simulink model "Exercicio_1f_sim"  (R2016a)
settings: Solver=VariableStepAuto  StartTime=0.0  StopTime=t_sim  RelTol=1e-3
values from neighbouring files (symbols this model uses):
  A = [[0,1,0];[0,0,1];[-0.005,-0.11,-0.7]]    [Exercicio_1.m]    (also in matlab.mat = [0  1  0; 0  0  1; -0.005  0.11  -0.7])
  A2 = [[-0.2,-0.2,0.4];[0.5,0,1];[0,-0.4,-0.4]]    [Exercicio_1.m]    (also in matlab.mat = [-0.2  -0.2  0.4; 0.5  0  1; 0  -0.4  -0.4])
  A_AObs = (A_Abb-(A_Ke*A_Aab))    [Exercicio_1.m]    (also in Exercicio_1_teste.m)
  A_BObs = ((A_AObs*A_Ke) + A_Aba - (A_Ke*A_Aaa))    [Exercicio_1.m]    (also in Exercicio_1_teste.m = ((A_AObs*Ke) + A_Aba - (A_Ke*A_Aaa)))
  A_CObs = [[0 0];[eye(2)]]    [Exercicio_1.m]    (also in Exercicio_1_teste.m = (eye(2)))
  A_DObs = [1;A_Ke]    [Exercicio_1.m]    (also in Exercicio_1_teste.m)
  A_FObs = (A_Bb - (A_Ke*A_Ba))    [Exercicio_1.m]    (also in Exercicio_1_teste.m)
  A_K_cntrl = acker(A,B, p_mf)    [Exercicio_1.m]
  B = [[0.1];[-0.2];[-0.1]]    [Exercicio_1.m]    (also in matlab.mat = [0.1 -0.2 -0.1])
  B2 = [[0.01];[0];[0.05]]    [Exercicio_1.m]    (also in matlab.mat = [0.01 0 0.05])
  B_AObs = (B_Abb-(B_Ke*B_Aab))    [Exercicio_1.m]
  B_BObs = ((B_AObs*B_Ke) + B_Aba - (B_Ke*B_Aaa))    [Exercicio_1.m]
  B_CObs = [[0 0];[eye(2)]]    [Exercicio_1.m]
  B_DObs = [1;B_Ke]    [Exercicio_1.m]
  B_FObs = (B_Bb - (B_Ke*B_Ba))    [Exercicio_1.m]
  B_K_cntrl = acker(A2,B2, p_mfB)    [Exercicio_1.m]
  C = [0,0,1]    [Exercicio_1.m]    (also in matlab.mat = [0 0 1])
  C2 = [1,0,0]    [Exercicio_1.m]    (also in matlab.mat = [1 0 0])
  D = [0]    [Exercicio_1.m]    (also in matlab.mat = 0)
  D2 = [0]    [Exercicio_1.m]    (also in matlab.mat = 0)
  N_termo_A1f = rscale(AreordA,AreordB,AreordC,D,A_K_cntrl)    [Exercicio_1.m]
  N_termo_B1f = rscale(Breord,B2,C2,D2,B_K_cntrl)    [Exercicio_1.m]
settings Model: Creator=Usuario  LastModifiedBy=Eletrônica Auto Poli

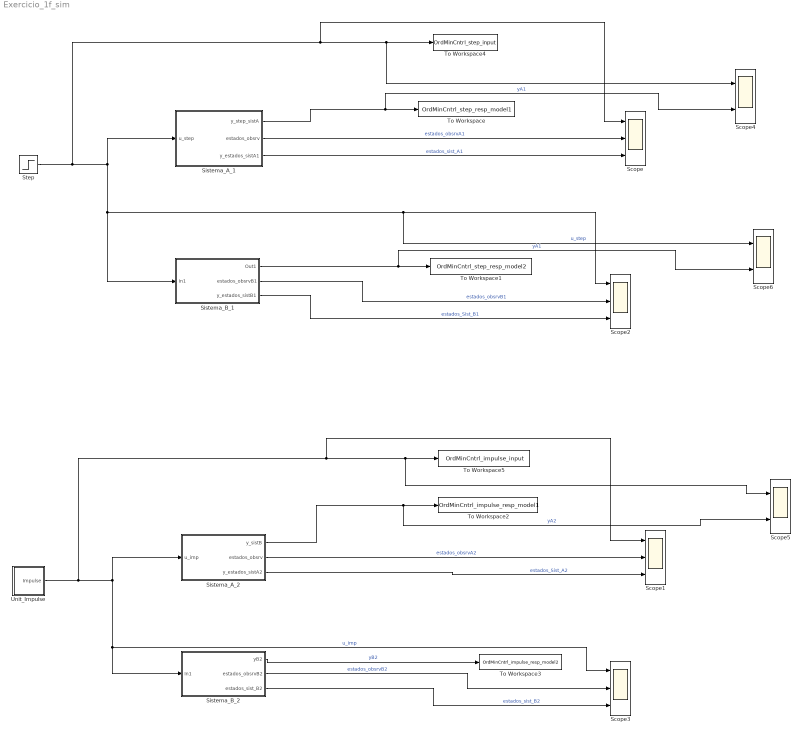
== system Exercicio_1f_sim ==
  Scope{,1..3} (4 alike) : Scope  NumInputPorts=3
  Scope4 : Scope  NumInputPorts=2
  Scope5 : Scope  NumInputPorts=2
  Scope6 : Scope  NumInputPorts=2
  Sistema_A_1 : Subsystem
  Sistema_A_2 : Subsystem
  Sistema_B_1 : Subsystem
  Sistema_B_2 : Subsystem
  Step : Step  SampleTime=0.01
  To Workspace : ToWorkspace  VariableName=OrdMinCntrl_step_resp_model1  SaveFormat=Timeseries  SampleTime=-1
  To Workspace1 : ToWorkspace  VariableName=OrdMinCntrl_step_resp_model2  SaveFormat=Timeseries  SampleTime=-1
  To Workspace2 : ToWorkspace  VariableName=OrdMinCntrl_impulse_resp_model1  SaveFormat=Timeseries  SampleTime=-1
  To Workspace3 : ToWorkspace  VariableName=OrdMinCntrl_impulse_resp_model2  SaveFormat=Timeseries  SampleTime=-1
  To Workspace4 : ToWorkspace  VariableName=OrdMinCntrl_step_input  SaveFormat=Timeseries  SampleTime=-1
  To Workspace5 : ToWorkspace  VariableName=OrdMinCntrl_impulse_input  SaveFormat=Timeseries  SampleTime=-1
  Unit_Impulse : Subsystem
  wires:
  Sistema_A_1/1(y_step_sistA) -> Scope4/2, To Workspace/1  "yA1"
  Sistema_A_1/2(estados_obsrv) -> Scope/2  "estados_obsrvA1"
  Unit_Impulse/1(Impulse) -> Scope1/1, Scope5/1, To Workspace5/1, Sistema_A_2/1(u_imp), Sistema_B_2/1(In1), Scope3/1  "u_imp"
  Sistema_A_2/1(y_sistB) -> Scope5/2, To Workspace2/1  "yA2"
  Sistema_B_2/1(yB2) -> To Workspace3/1  "yB2"
  Sistema_A_2/2(estados_obsrv) -> Scope1/2  "estados_obsrvA2"
  Sistema_B_1/2(estados_obsrvB1) -> Scope2/2  "estados_obsrvB1"
  Sistema_B_2/2(estados_obsrvB2) -> Scope3/2  "estados_obsrvB2"
  Sistema_A_2/3(y_estados_sistA2) -> Scope1/3  "estados_Sist_A2"
  Sistema_B_2/3(estados_sist_B2) -> Scope3/3  "estados_sist_B2"
  Sistema_B_1/3(y_estados_sistB1) -> Scope2/3  "estados_Sist_B1"
  Sistema_A_1/3(y_estados_sistA1) -> Scope/3  "estados_sist_A1"
  Step/1 -> Scope/1, Scope4/1, To Workspace4/1, Sistema_A_1/1(u_step), Scope6/1, Scope2/1, Sistema_B_1/1(In1)  "u_step"
  Sistema_B_1/1(Out1) -> Scope6/2, To Workspace1/1  "yA1"

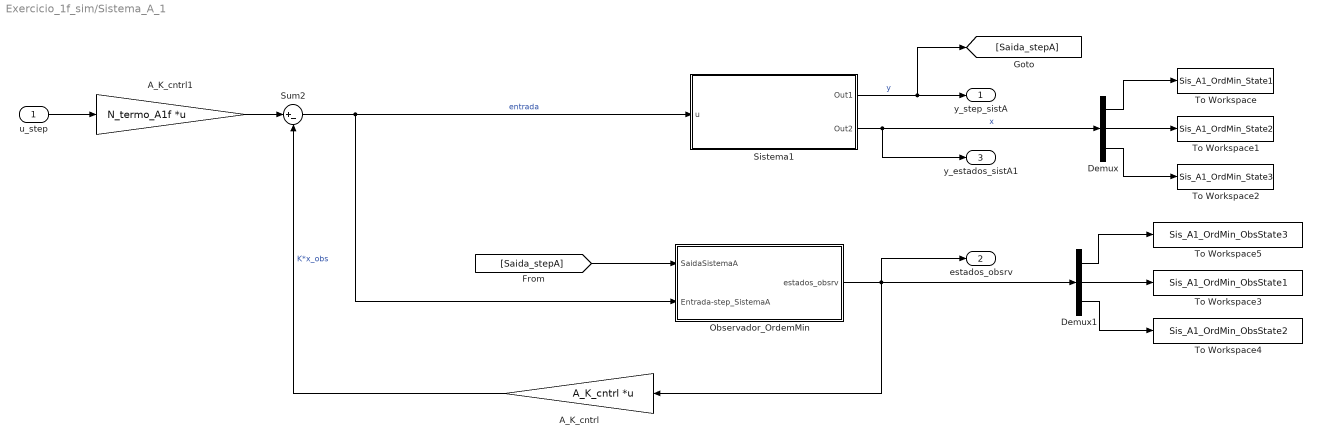
== system Exercicio_1f_sim/Sistema_A_1 ==
  u_step : Inport
  A_K_cntrl : Gain  Gain=A_K_cntrl  Multiplication=Matrix(K*u)
  A_K_cntrl1 : Gain  Gain=N_termo_A1f  Multiplication=Matrix(K*u)
  Demux : Demux  Outputs=3
  Demux1 : Demux  Outputs=3
  Observador_OrdemMin : Subsystem
  Sistema1 : Subsystem
  Sum2 : Sum  Inputs=|+-
  To Workspace : ToWorkspace  VariableName=Sis_A1_OrdMin_State1  SaveFormat=Timeseries  SampleTime=-1
  To Workspace1 : ToWorkspace  VariableName=Sis_A1_OrdMin_State2  SaveFormat=Timeseries  SampleTime=-1
  To Workspace2 : ToWorkspace  VariableName=Sis_A1_OrdMin_State3  SaveFormat=Timeseries  SampleTime=-1
  To Workspace3 : ToWorkspace  VariableName=Sis_A1_OrdMin_ObsState1  SaveFormat=Timeseries  SampleTime=-1
  To Workspace4 : ToWorkspace  VariableName=Sis_A1_OrdMin_ObsState2  SaveFormat=Timeseries  SampleTime=-1
  To Workspace5 : ToWorkspace  VariableName=Sis_A1_OrdMin_ObsState3  SaveFormat=Timeseries  SampleTime=-1
  y_step_sistA : Outport
  estados_obsrv : Outport  Port=2
  y_estados_sistA1 : Outport  Port=3
  wires:
  Demux/1 -> To Workspace/1
  Demux/2 -> To Workspace1/1
  Demux/3 -> To Workspace2/1
  Sum2/1 -> Sistema1/1(u), Observador_OrdemMin/2(Entrada-step_SistemaA)  "entrada"
  Sistema1/1(Out1) -> [Saida_stepA], y_step_sistA/1  "y"
  Sistema1/2(Out2) -> y_estados_sistA1/1, Demux/1  "x"
  Demux1/1 -> To Workspace5/1
  Demux1/2 -> To Workspace3/1
  Demux1/3 -> To Workspace4/1
  Observador_OrdemMin/1(estados_obsrv) -> Demux1/1, A_K_cntrl/1, estados_obsrv/1
  [Saida_stepA] -> Observador_OrdemMin/1(SaidaSistemaA)
  A_K_cntrl/1 -> Sum2/2  "K*x_obs"
  u_step/1 -> A_K_cntrl1/1
  A_K_cntrl1/1 -> Sum2/1

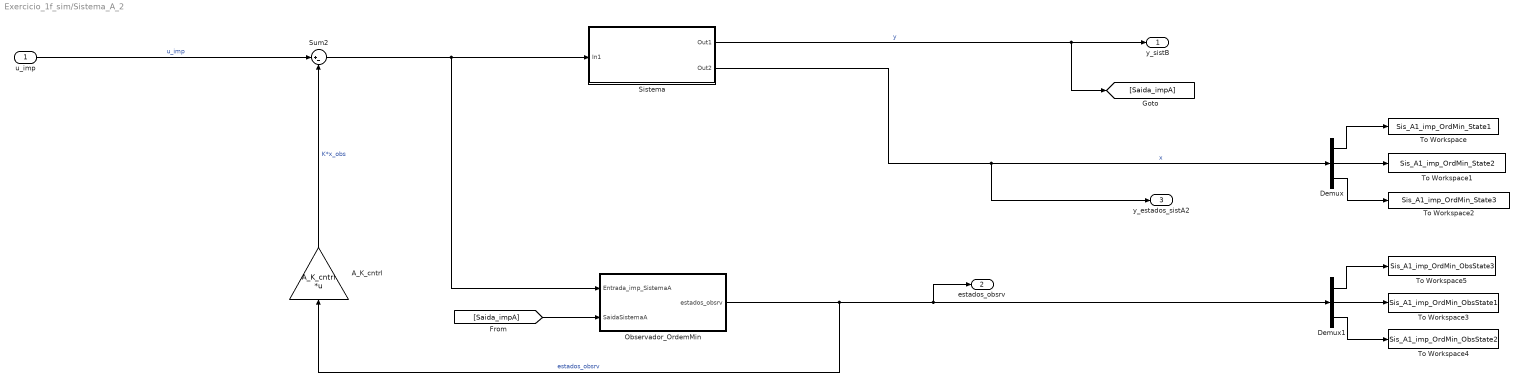
== system Exercicio_1f_sim/Sistema_A_2 ==
  u_imp : Inport
  A_K_cntrl : Gain  Gain=A_K_cntrl  Multiplication=Matrix(K*u)
  Demux : Demux  Outputs=3
  Demux1 : Demux  Outputs=3
  Observador_OrdemMin : Subsystem
  Sistema : Subsystem
  Sum2 : Sum  Inputs=|+-
  To Workspace : ToWorkspace  VariableName=Sis_A1_imp_OrdMin_State1  SaveFormat=Timeseries  SampleTime=-1
  To Workspace1 : ToWorkspace  VariableName=Sis_A1_imp_OrdMin_State2  SaveFormat=Timeseries  SampleTime=-1
  To Workspace2 : ToWorkspace  VariableName=Sis_A1_imp_OrdMin_State3  SaveFormat=Timeseries  SampleTime=-1
  To Workspace3 : ToWorkspace  VariableName=Sis_A1_imp_OrdMin_ObsState1  SaveFormat=Timeseries  SampleTime=-1
  To Workspace4 : ToWorkspace  VariableName=Sis_A1_imp_OrdMin_ObsState2  SaveFormat=Timeseries  SampleTime=-1
  To Workspace5 : ToWorkspace  VariableName=Sis_A1_imp_OrdMin_ObsState3  SaveFormat=Timeseries  SampleTime=-1
  y_sistB : Outport
  estados_obsrv : Outport  Port=2
  y_estados_sistA2 : Outport  Port=3
  wires:
  Demux/1 -> To Workspace/1
  Demux/2 -> To Workspace1/1
  Demux/3 -> To Workspace2/1
  Sum2/1 -> Sistema/1(In1), Observador_OrdemMin/1(Entrada_imp_SistemaA)
  Demux1/1 -> To Workspace5/1
  Demux1/2 -> To Workspace3/1
  Demux1/3 -> To Workspace4/1
  Observador_OrdemMin/1(estados_obsrv) -> A_K_cntrl/1, estados_obsrv/1, Demux1/1  "estados_obsrv"
  Sistema/2(Out2) -> y_estados_sistA2/1, Demux/1  "x"
  Sistema/1(Out1) -> [Saida_impA], y_sistB/1  "y"
  [Saida_impA] -> Observador_OrdemMin/2(SaidaSistemaA)
  A_K_cntrl/1 -> Sum2/2  "K*x_obs"
  u_imp/1 -> Sum2/1  "u_imp"

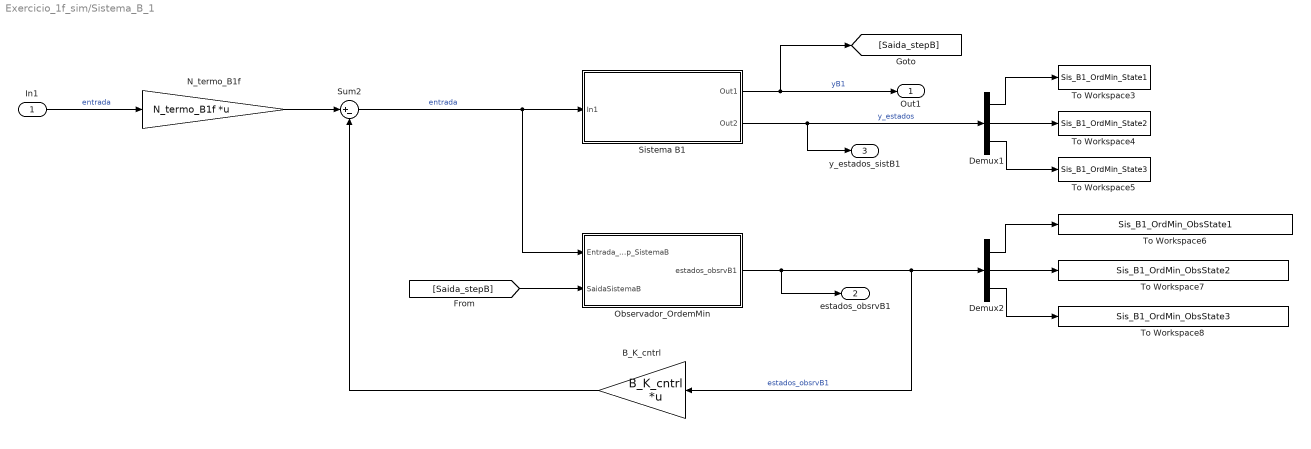
== system Exercicio_1f_sim/Sistema_B_1 ==
  In1 : Inport
  B_K_cntrl : Gain  Gain=B_K_cntrl  Multiplication=Matrix(K*u)
  Demux1 : Demux  Outputs=3
  Demux2 : Demux  Outputs=3
  N_termo_B1f : Gain  Gain=N_termo_B1f  Multiplication=Matrix(K*u)
  Observador_OrdemMin : Subsystem
  Sistema B1 : Subsystem
  Sum2 : Sum  Inputs=|+-
  To Workspace3 : ToWorkspace  VariableName=Sis_B1_OrdMin_State1  SaveFormat=Timeseries  SampleTime=-1
  To Workspace4 : ToWorkspace  VariableName=Sis_B1_OrdMin_State2  SaveFormat=Timeseries  SampleTime=-1
  To Workspace5 : ToWorkspace  VariableName=Sis_B1_OrdMin_State3  SaveFormat=Timeseries  SampleTime=-1
  To Workspace6 : ToWorkspace  VariableName=Sis_B1_OrdMin_ObsState1  SaveFormat=Timeseries  SampleTime=-1
  To Workspace7 : ToWorkspace  VariableName=Sis_B1_OrdMin_ObsState2  SaveFormat=Timeseries  SampleTime=-1
  To Workspace8 : ToWorkspace  VariableName=Sis_B1_OrdMin_ObsState3  SaveFormat=Timeseries  SampleTime=-1
  Out1 : Outport
  estados_obsrvB1 : Outport  Port=2
  y_estados_sistB1 : Outport  Port=3
  wires:
  Demux1/1 -> To Workspace3/1
  Demux1/2 -> To Workspace4/1
  Demux1/3 -> To Workspace5/1
  Sum2/1 -> Observador_OrdemMin/1(Entrada_step_SistemaB), Sistema B1/1(In1)  "entrada"
  Sistema B1/1(Out1) -> [Saida_stepB], Out1/1  "yB1"
  Demux2/1 -> To Workspace6/1
  Demux2/2 -> To Workspace7/1
  Demux2/3 -> To Workspace8/1
  Observador_OrdemMin/1(estados_obsrvB1) -> Demux2/1, B_K_cntrl/1, estados_obsrvB1/1  "estados_obsrvB1"
  Sistema B1/2(Out2) -> y_estados_sistB1/1, Demux1/1  "y_estados"
  [Saida_stepB] -> Observador_OrdemMin/2(SaidaSistemaB)
  In1/1 -> N_termo_B1f/1  "entrada"
  B_K_cntrl/1 -> Sum2/2
  N_termo_B1f/1 -> Sum2/1

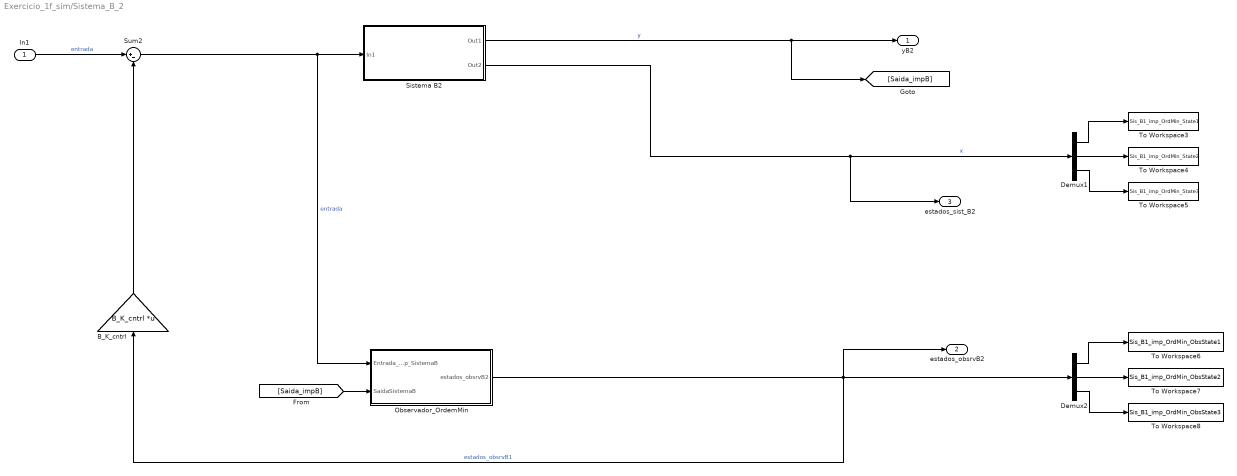
== system Exercicio_1f_sim/Sistema_B_2 ==
  In1 : Inport
  B_K_cntrl : Gain  Gain=B_K_cntrl  Multiplication=Matrix(K*u)
  Demux1 : Demux  Outputs=3
  Demux2 : Demux  Outputs=3
  Observador_OrdemMin : Subsystem
  Sistema B2 : Subsystem
  Sum2 : Sum  Inputs=|+-
  To Workspace3 : ToWorkspace  VariableName=Sis_B1_imp_OrdMin_State1  SaveFormat=Timeseries  SampleTime=-1
  To Workspace4 : ToWorkspace  VariableName=Sis_B1_imp_OrdMin_State2  SaveFormat=Timeseries  SampleTime=-1
  To Workspace5 : ToWorkspace  VariableName=Sis_B1_imp_OrdMin_State3  SaveFormat=Timeseries  SampleTime=-1
  To Workspace6 : ToWorkspace  VariableName=Sis_B1_imp_OrdMin_ObsState1  SaveFormat=Timeseries  SampleTime=-1
  To Workspace7 : ToWorkspace  VariableName=Sis_B1_imp_OrdMin_ObsState2  SaveFormat=Timeseries  SampleTime=-1
  To Workspace8 : ToWorkspace  VariableName=Sis_B1_imp_OrdMin_ObsState3  SaveFormat=Timeseries  SampleTime=-1
  yB2 : Outport
  estados_obsrvB2 : Outport  Port=2
  estados_sist_B2 : Outport  Port=3
  wires:
  Demux1/1 -> To Workspace3/1
  Demux1/2 -> To Workspace4/1
  Demux1/3 -> To Workspace5/1
  Sum2/1 -> Observador_OrdemMin/1(Entrada_step_SistemaB), Sistema B2/1(In1)  "entrada"
  Sistema B2/1(Out1) -> [Saida_impB], yB2/1  "y"
  Demux2/1 -> To Workspace6/1
  Demux2/2 -> To Workspace7/1
  Demux2/3 -> To Workspace8/1
  Sistema B2/2(Out2) -> estados_sist_B2/1, Demux1/1  "x"
  Observador_OrdemMin/1(estados_obsrvB2) -> B_K_cntrl/1, estados_obsrvB2/1, Demux2/1  "estados_obsrvB1"
  In1/1 -> Sum2/1  "entrada"
  B_K_cntrl/1 -> Sum2/2
  [Saida_impB] -> Observador_OrdemMin/2(SaidaSistemaB)

== system Exercicio_1f_sim/Unit_Impulse ==
  Step1 : Step  Time=0.5  After=100  SampleTime=0.01
  Step2 : Step  Time=0.51  After=100  SampleTime=0.01
  Sum : Sum  Inputs=|+-
  Impulse : Outport
  wires:
  Step2/1 -> Sum/2
  Step1/1 -> Sum/1
  Sum/1 -> Impulse/1

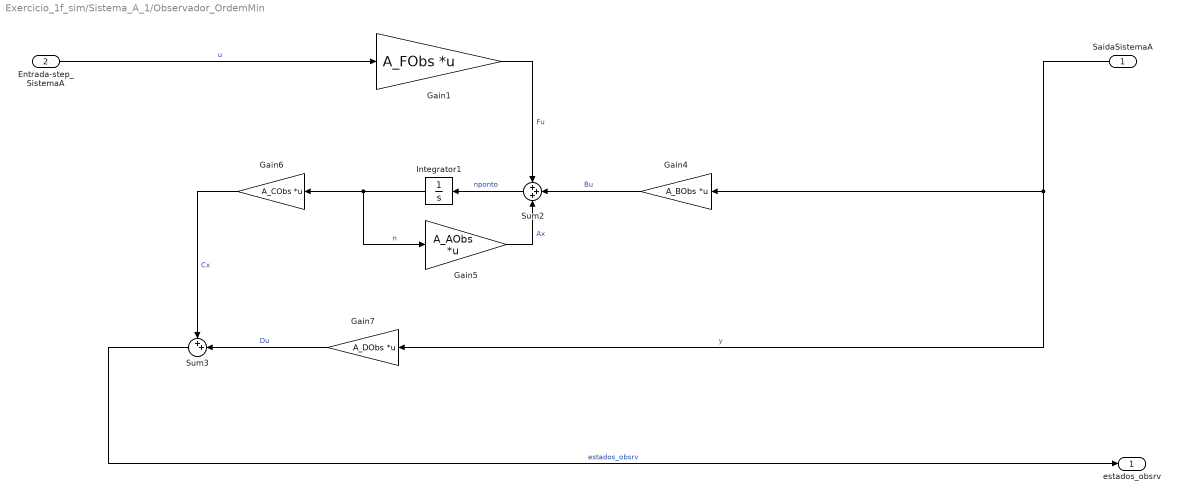
== system Exercicio_1f_sim/Sistema_A_1/Observador_OrdemMin ==
  SaidaSistemaA : Inport
  Entrada-step_SistemaA : Inport  Port=2
  Gain1 : Gain  Gain=A_FObs  Multiplication=Matrix(K*u)
  Gain4 : Gain  Gain=A_BObs  Multiplication=Matrix(K*u)
  Gain5 : Gain  Gain=A_AObs  Multiplication=Matrix(K*u)
  Gain6 : Gain  Gain=A_CObs  Multiplication=Matrix(K*u)
  Gain7 : Gain  Gain=A_DObs  Multiplication=Matrix(K*u)
  Integrator1 : Integrator  UpperSaturationLimit=1.279387983436996e+55  LowerSaturationLimit=0
  Sum2 : Sum  Inputs=+++
  Sum3 : Sum  Inputs=++|
  estados_obsrv : Outport
  wires:
  Integrator1/1 -> Gain5/1, Gain6/1  "n"
  Gain6/1 -> Sum3/1  "Cx"
  SaidaSistemaA/1 -> Gain4/1, Gain7/1  "y"
  Sum3/1 -> estados_obsrv/1  "estados_obsrv"
  Gain7/1 -> Sum3/2  "Du"
  Gain4/1 -> Sum2/2  "Bu"
  Gain5/1 -> Sum2/3  "Ax"
  Gain1/1 -> Sum2/1  "Fu"
  Sum2/1 -> Integrator1/1  "nponto"
  Entrada-step_SistemaA/1 -> Gain1/1  "u"

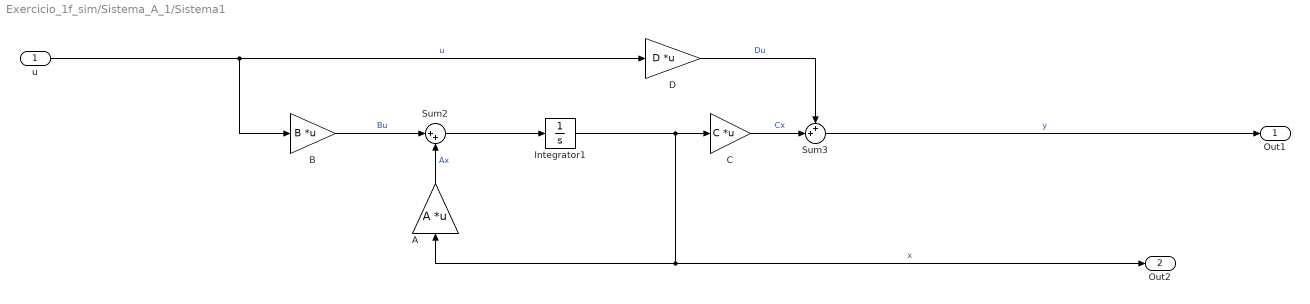
== system Exercicio_1f_sim/Sistema_A_1/Sistema1 ==
  u : Inport
  A : Gain  Gain=A  Multiplication=Matrix(K*u)
  B : Gain  Gain=B  Multiplication=Matrix(K*u)
  C : Gain  Gain=C  Multiplication=Matrix(K*u)
  D : Gain  Gain=D  Multiplication=Matrix(K*u)
  Integrator1 : Integrator
  Sum2 : Sum  Inputs=|++
  Sum3 : Sum  Inputs=++|
  Out1 : Outport
  Out2 : Outport  Port=2
  wires:
  u/1 -> B/1, D/1  "u"
  Sum3/1 -> Out1/1  "y"
  Integrator1/1 -> Out2/1, A/1, C/1  "x"
  C/1 -> Sum3/2  "Cx"
  D/1 -> Sum3/1  "Du"
  B/1 -> Sum2/1  "Bu"
  A/1 -> Sum2/2  "Ax"
  Sum2/1 -> Integrator1/1

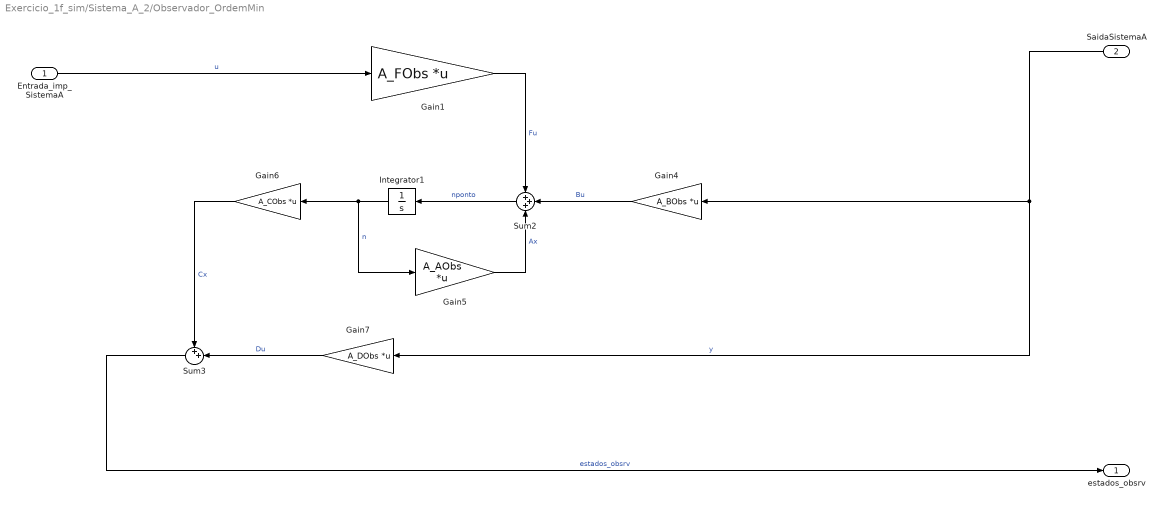
== system Exercicio_1f_sim/Sistema_A_2/Observador_OrdemMin ==
  Entrada_imp_SistemaA : Inport
  SaidaSistemaA : Inport  Port=2
  Gain1 : Gain  Gain=A_FObs  Multiplication=Matrix(K*u)
  Gain4 : Gain  Gain=A_BObs  Multiplication=Matrix(K*u)
  Gain5 : Gain  Gain=A_AObs  Multiplication=Matrix(K*u)
  Gain6 : Gain  Gain=A_CObs  Multiplication=Matrix(K*u)
  Gain7 : Gain  Gain=A_DObs  Multiplication=Matrix(K*u)
  Integrator1 : Integrator  UpperSaturationLimit=1.279387983436996e+55  LowerSaturationLimit=0
  Sum2 : Sum  Inputs=+++
  Sum3 : Sum  Inputs=++|
  estados_obsrv : Outport
  wires:
  Integrator1/1 -> Gain5/1, Gain6/1  "n"
  Gain6/1 -> Sum3/1  "Cx"
  SaidaSistemaA/1 -> Gain4/1, Gain7/1  "y"
  Sum3/1 -> estados_obsrv/1  "estados_obsrv"
  Gain7/1 -> Sum3/2  "Du"
  Gain4/1 -> Sum2/2  "Bu"
  Gain5/1 -> Sum2/3  "Ax"
  Gain1/1 -> Sum2/1  "Fu"
  Sum2/1 -> Integrator1/1  "nponto"
  Entrada_imp_SistemaA/1 -> Gain1/1  "u"

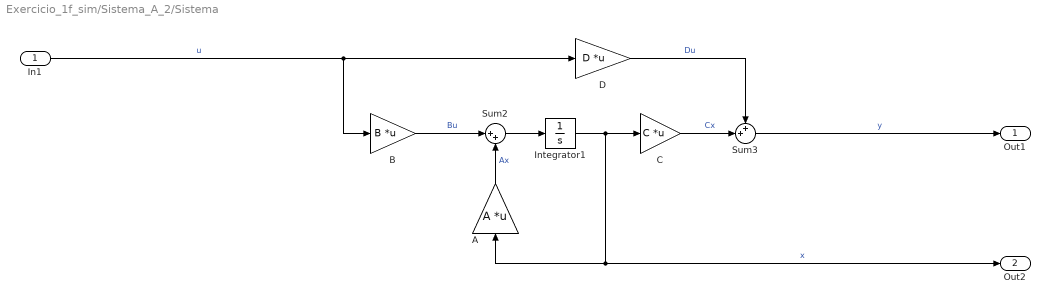
== system Exercicio_1f_sim/Sistema_A_2/Sistema ==
  In1 : Inport
  A : Gain  Gain=A  Multiplication=Matrix(K*u)
  B : Gain  Gain=B  Multiplication=Matrix(K*u)
  C : Gain  Gain=C  Multiplication=Matrix(K*u)
  D : Gain  Gain=D  Multiplication=Matrix(K*u)
  Integrator1 : Integrator
  Sum2 : Sum  Inputs=|++
  Sum3 : Sum  Inputs=++|
  Out1 : Outport
  Out2 : Outport  Port=2
  wires:
  In1/1 -> B/1, D/1  "u"
  Sum3/1 -> Out1/1  "y"
  Integrator1/1 -> Out2/1, A/1, C/1  "x"
  C/1 -> Sum3/2  "Cx"
  D/1 -> Sum3/1  "Du"
  B/1 -> Sum2/1  "Bu"
  A/1 -> Sum2/2  "Ax"
  Sum2/1 -> Integrator1/1

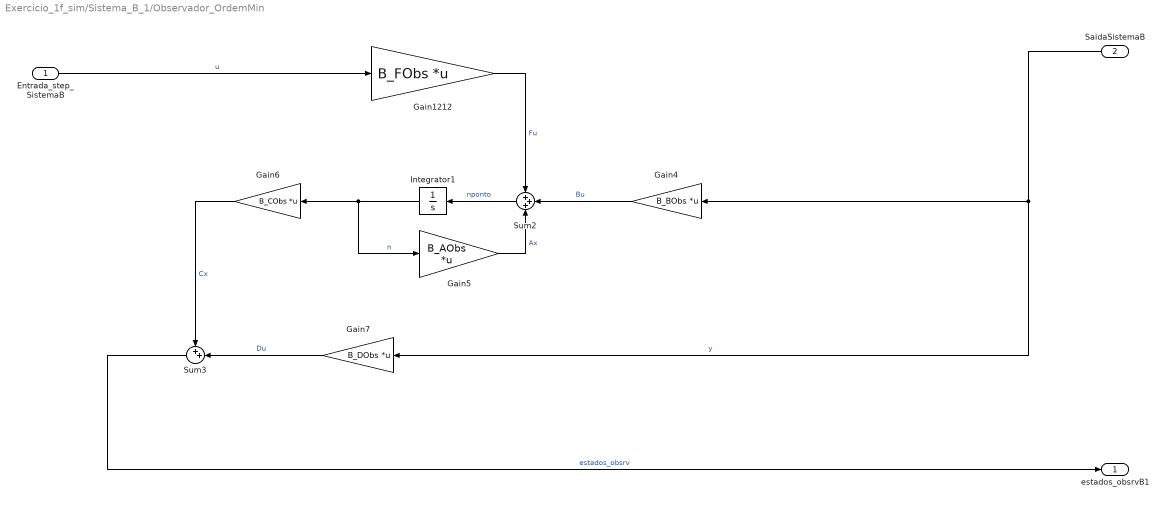
== system Exercicio_1f_sim/Sistema_B_1/Observador_OrdemMin ==
  Entrada_step_SistemaB : Inport
  SaidaSistemaB : Inport  Port=2
  Gain1212 : Gain  Gain=B_FObs  Multiplication=Matrix(K*u)
  Gain4 : Gain  Gain=B_BObs  Multiplication=Matrix(K*u)
  Gain5 : Gain  Gain=B_AObs  Multiplication=Matrix(K*u)
  Gain6 : Gain  Gain=B_CObs  Multiplication=Matrix(K*u)
  Gain7 : Gain  Gain=B_DObs  Multiplication=Matrix(K*u)
  Integrator1 : Integrator
  Sum2 : Sum  Inputs=+++
  Sum3 : Sum  Inputs=++|
  estados_obsrvB1 : Outport
  wires:
  Integrator1/1 -> Gain5/1, Gain6/1  "n"
  Gain6/1 -> Sum3/1  "Cx"
  SaidaSistemaB/1 -> Gain4/1, Gain7/1  "y"
  Sum3/1 -> estados_obsrvB1/1  "estados_obsrv"
  Gain7/1 -> Sum3/2  "Du"
  Gain4/1 -> Sum2/2  "Bu"
  Gain5/1 -> Sum2/3  "Ax"
  Sum2/1 -> Integrator1/1  "nponto"
  Entrada_step_SistemaB/1 -> Gain1212/1  "u"
  Gain1212/1 -> Sum2/1  "Fu"

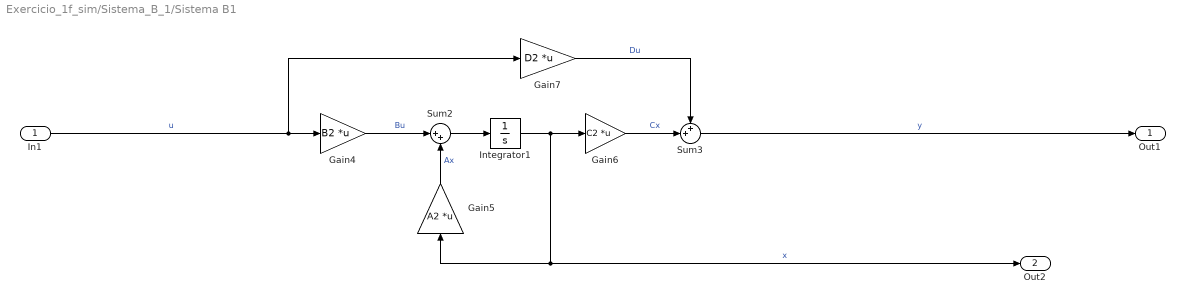
== system Exercicio_1f_sim/Sistema_B_1/Sistema B1 ==
  In1 : Inport
  Gain4 : Gain  Gain=B2  Multiplication=Matrix(K*u)
  Gain5 : Gain  Gain=A2  Multiplication=Matrix(K*u)
  Gain6 : Gain  Gain=C2  Multiplication=Matrix(K*u)
  Gain7 : Gain  Gain=D2  Multiplication=Matrix(K*u)
  Integrator1 : Integrator
  Sum2 : Sum  Inputs=|++
  Sum3 : Sum  Inputs=++|
  Out1 : Outport
  Out2 : Outport  Port=2
  wires:
  In1/1 -> Gain7/1, Gain4/1  "u"
  Sum3/1 -> Out1/1  "y"
  Integrator1/1 -> Out2/1, Gain5/1, Gain6/1  "x"
  Gain6/1 -> Sum3/2  "Cx"
  Gain7/1 -> Sum3/1  "Du"
  Gain4/1 -> Sum2/1  "Bu"
  Gain5/1 -> Sum2/2  "Ax"
  Sum2/1 -> Integrator1/1

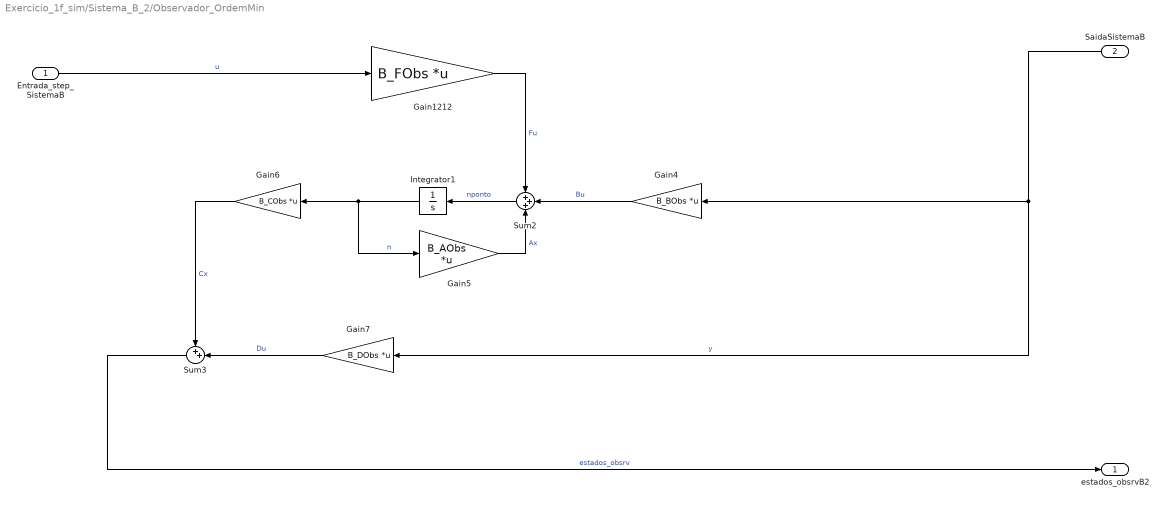
== system Exercicio_1f_sim/Sistema_B_2/Observador_OrdemMin ==
  Entrada_step_SistemaB : Inport
  SaidaSistemaB : Inport  Port=2
  Gain1212 : Gain  Gain=B_FObs  Multiplication=Matrix(K*u)
  Gain4 : Gain  Gain=B_BObs  Multiplication=Matrix(K*u)
  Gain5 : Gain  Gain=B_AObs  Multiplication=Matrix(K*u)
  Gain6 : Gain  Gain=B_CObs  Multiplication=Matrix(K*u)
  Gain7 : Gain  Gain=B_DObs  Multiplication=Matrix(K*u)
  Integrator1 : Integrator  InitialCondition=[10 21]
  Sum2 : Sum  Inputs=+++
  Sum3 : Sum  Inputs=++|
  estados_obsrvB2 : Outport
  wires:
  Integrator1/1 -> Gain5/1, Gain6/1  "n"
  Gain6/1 -> Sum3/1  "Cx"
  SaidaSistemaB/1 -> Gain4/1, Gain7/1  "y"
  Sum3/1 -> estados_obsrvB2/1  "estados_obsrv"
  Gain7/1 -> Sum3/2  "Du"
  Gain4/1 -> Sum2/2  "Bu"
  Gain5/1 -> Sum2/3  "Ax"
  Sum2/1 -> Integrator1/1  "nponto"
  Entrada_step_SistemaB/1 -> Gain1212/1  "u"
  Gain1212/1 -> Sum2/1  "Fu"

== system Exercicio_1f_sim/Sistema_B_2/Sistema B2 ==
  In1 : Inport
  Gain4 : Gain  Gain=B2  Multiplication=Matrix(K*u)
  Gain5 : Gain  Gain=A2  Multiplication=Matrix(K*u)
  Gain6 : Gain  Gain=C2  Multiplication=Matrix(K*u)
  Gain7 : Gain  Gain=D2  Multiplication=Matrix(K*u)
  Integrator1 : Integrator
  Sum2 : Sum  Inputs=|++
  Sum3 : Sum  Inputs=++|
  Out1 : Outport
  Out2 : Outport  Port=2
  wires:
  In1/1 -> Gain7/1, Gain4/1  "u"
  Sum3/1 -> Out1/1  "y"
  Integrator1/1 -> Out2/1, Gain5/1, Gain6/1  "x"
  Gain6/1 -> Sum3/2  "Cx"
  Gain7/1 -> Sum3/1  "Du"
  Gain4/1 -> Sum2/1  "Bu"
  Gain5/1 -> Sum2/2  "Ax"
  Sum2/1 -> Integrator1/1
